simulink model "dc_motor_sim"  (R2017a)
settings: Solver=FixedStepAuto  StartTime=0.0  StopTime=0.5  FixedStep=1e-4  RelTol=1e-3
InitFcn:
  | Tw=0.02;     %Ancho de Ventana.
  | ppv=20;      %Pulsos por vuelta.
  | Ts=1e-4;     %Tiempo de muestreo.
settings Model: Creator=Martin  LastModifiedBy=Martin

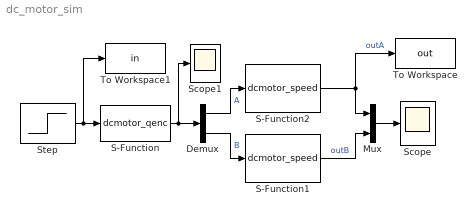
== system dc_motor_sim ==
  Demux : Demux  Outputs=2
  Mux : Mux  Inputs=2
  S-Function : S-Function  FunctionName=dcmotor_qenc  Parameters=ppv  SFunctionDeploymentMode=off  EnableBusSupport=off
  S-Function1 : S-Function  FunctionName=dcmotor_speed  Parameters=Ts,ppv,Tw  SFunctionDeploymentMode=off  EnableBusSupport=off
  S-Function2 : S-Function  FunctionName=dcmotor_speed  Parameters=Ts,ppv,Tw  SFunctionDeploymentMode=off  EnableBusSupport=off
  Scope : Scope
  Scope1 : Scope
  Step : Step  Time=0  After=12  SampleTime=Ts
  To Workspace : ToWorkspace  VariableName=out  SaveFormat=Timeseries  SampleTime=Tw
  To Workspace1 : ToWorkspace  VariableName=in  SaveFormat=Timeseries  SampleTime=Tw
  wires:
  Step/1 -> To Workspace1/1, S-Function/1
  S-Function/1 -> Scope1/1, Demux/1
  Demux/2 -> S-Function1/1  "B"
  Demux/1 -> S-Function2/1  "A"
  Mux/1 -> Scope/1
  S-Function2/1 -> To Workspace/1, Mux/1  "outA"
  S-Function1/1 -> Mux/2  "outB"
